simulink model "FullCarLateral"  (R2023b)
settings: Solver=FixedStepAuto  StartTime=0.0  StopTime=30  FixedStep=dt  MaxStep=0.001  RelTol=1e-3
model workspace (MAT data in the model file):
  AMU : Simulink.Signal (value not decoded)
  EPSILON : Simulink.Signal (value not decoded)
  FZO : Simulink.Signal (value not decoded)
  LCX : Simulink.Signal (value not decoded)
  LCY : Simulink.Signal (value not decoded)
  LCZ : Simulink.Signal (value not decoded)
  LEX : Simulink.Signal (value not decoded)
  LEY : Simulink.Signal (value not decoded)
  LFZO : Simulink.Signal (value not decoded)
  LHX : Simulink.Signal (value not decoded)
  LHY : Simulink.Signal (value not decoded)
  LKXKAPPA : Simulink.Signal (value not decoded)
  LKYALPHA : Simulink.Signal (value not decoded)
  LKYGAMMA : Simulink.Signal (value not decoded)
  LKZGAMMA : Simulink.Signal (value not decoded)
  LMR : Simulink.Signal (value not decoded)
  LMUV : Simulink.Signal (value not decoded)
  LMUX : Simulink.Signal (value not decoded)
  LMUXAST : Simulink.Signal (value not decoded)
  LMUXPRIME : Simulink.Signal (value not decoded)
  LMUY : Simulink.Signal (value not decoded)
  LMUYAST : Simulink.Signal (value not decoded)
  LMUYPRIME : Simulink.Signal (value not decoded)
  LMX : Simulink.Signal (value not decoded)
  LMY : Simulink.Signal (value not decoded)
  LS : Simulink.Signal (value not decoded)
  LT : Simulink.Signal (value not decoded)
  LVX : Simulink.Signal (value not decoded)
  LVY : Simulink.Signal (value not decoded)
  LVYKAPPA : Simulink.Signal (value not decoded)
  LXALPHA : Simulink.Signal (value not decoded)
  LYKAPPA : Simulink.Signal (value not decoded)
  PCX1 : Simulink.Signal (value not decoded)
  PCY1 : Simulink.Signal (value not decoded)
  PDX1 : Simulink.Signal (value not decoded)
  PDX2 : Simulink.Signal (value not decoded)
  PDX3 : Simulink.Signal (value not decoded)
  PDY1 : Simulink.Signal (value not decoded)
  PDY2 : Simulink.Signal (value not decoded)
  PDY3 : Simulink.Signal (value not decoded)
  PEX1 : Simulink.Signal (value not decoded)
  PEX2 : Simulink.Signal (value not decoded)
  PEX3 : Simulink.Signal (value not decoded)
  PEX4 : Simulink.Signal (value not decoded)
  PEY1 : Simulink.Signal (value not decoded)
  PEY2 : Simulink.Signal (value not decoded)
  PEY3 : Simulink.Signal (value not decoded)
  PEY4 : Simulink.Signal (value not decoded)
  PEY5 : Simulink.Signal (value not decoded)
  PHX1 : Simulink.Signal (value not decoded)
  PHX2 : Simulink.Signal (value not decoded)
  PHY1 : Simulink.Signal (value not decoded)
  PHY2 : Simulink.Signal (value not decoded)
  PKX1 : Simulink.Signal (value not decoded)
  PKX2 : Simulink.Signal (value not decoded)
  PKX3 : Simulink.Signal (value not decoded)
  PKY1 : Simulink.Signal (value not decoded)
  PKY2 : Simulink.Signal (value not decoded)
  PKY3 : Simulink.Signal (value not decoded)
  PKY4 : Simulink.Signal (value not decoded)
  PKY5 : Simulink.Signal (value not decoded)
  PKY6 : Simulink.Signal (value not decoded)
  PKY7 : Simulink.Signal (value not decoded)
  PVX1 : Simulink.Signal (value not decoded)
  PVX2 : Simulink.Signal (value not decoded)
  PVY1 : Simulink.Signal (value not decoded)
  PVY2 : Simulink.Signal (value not decoded)
  PVY3 : Simulink.Signal (value not decoded)
  PVY4 : Simulink.Signal (value not decoded)
  QBZ1 : Simulink.Signal (value not decoded)
  QBZ10 : Simulink.Signal (value not decoded)
  QBZ2 : Simulink.Signal (value not decoded)
  QBZ3 : Simulink.Signal (value not decoded)
  QBZ5 : Simulink.Signal (value not decoded)
  QBZ6 : Simulink.Signal (value not decoded)
  QBZ9 : Simulink.Signal (value not decoded)
  QCZ1 : Simulink.Signal (value not decoded)
  QDZ1 : Simulink.Signal (value not decoded)
  QDZ10 : Simulink.Signal (value not decoded)
  QDZ11 : Simulink.Signal (value not decoded)
  QDZ2 : Simulink.Signal (value not decoded)
  QDZ3 : Simulink.Signal (value not decoded)
  QDZ4 : Simulink.Signal (value not decoded)
  QDZ6 : Simulink.Signal (value not decoded)
  QDZ7 : Simulink.Signal (value not decoded)
  QDZ8 : Simulink.Signal (value not decoded)
  QDZ9 : Simulink.Signal (value not decoded)
  QEZ1 : Simulink.Signal (value not decoded)
  QEZ2 : Simulink.Signal (value not decoded)
  QEZ3 : Simulink.Signal (value not decoded)
  QEZ4 : Simulink.Signal (value not decoded)
  QEZ5 : Simulink.Signal (value not decoded)
  QHZ1 : Simulink.Signal (value not decoded)
  QHZ2 : Simulink.Signal (value not decoded)
  QHZ3 : Simulink.Signal (value not decoded)
  QHZ4 : Simulink.Signal (value not decoded)
  QSX1 : Simulink.Signal (value not decoded)
  QSX2 : Simulink.Signal (value not decoded)
  QSX3 : Simulink.Signal (value not decoded)
  QX1 : Simulink.Signal (value not decoded)
  QX2 : Simulink.Signal (value not decoded)
  QX3 : Simulink.Signal (value not decoded)
  QX4 : Simulink.Signal (value not decoded)
  QX5 : Simulink.Signal (value not decoded)
  QX6 : Simulink.Signal (value not decoded)
  RBX1 : Simulink.Signal (value not decoded)
  RBX2 : Simulink.Signal (value not decoded)
  RBX3 : Simulink.Signal (value not decoded)
  RBY1 : Simulink.Signal (value not decoded)
  RBY2 : Simulink.Signal (value not decoded)
  RBY3 : Simulink.Signal (value not decoded)
  RBY4 : Simulink.Signal (value not decoded)
  RCX1 : Simulink.Signal (value not decoded)
  RCY1 : Simulink.Signal (value not decoded)
  REX1 : Simulink.Signal (value not decoded)
  REX2 : Simulink.Signal (value not decoded)
  REY1 : Simulink.Signal (value not decoded)
  REY2 : Simulink.Signal (value not decoded)
  RHX1 : Simulink.Signal (value not decoded)
  RHY1 : Simulink.Signal (value not decoded)
  RHY2 : Simulink.Signal (value not decoded)
  RO : Simulink.Signal (value not decoded)
  RVY1 : Simulink.Signal (value not decoded)
  RVY2 : Simulink.Signal (value not decoded)
  RVY3 : Simulink.Signal (value not decoded)
  RVY4 : Simulink.Signal (value not decoded)
  RVY5 : Simulink.Signal (value not decoded)
  RVY6 : Simulink.Signal (value not decoded)
  SSZ1 : Simulink.Signal (value not decoded)
  SSZ2 : Simulink.Signal (value not decoded)
  SSZ3 : Simulink.Signal (value not decoded)
  SSZ4 : Simulink.Signal (value not decoded)
  VCX : Simulink.Signal (value not decoded)
  ZETA0 : Simulink.Signal (value not decoded)
  ZETA1 : Simulink.Signal (value not decoded)
  ZETA2 : Simulink.Signal (value not decoded)
  ZETA3 : Simulink.Signal (value not decoded)
  ZETA4 : Simulink.Signal (value not decoded)
  ZETA5 : Simulink.Signal (value not decoded)
  ZETA6 : Simulink.Signal (value not decoded)
  ZETA7 : Simulink.Signal (value not decoded)
  ZETA8 : Simulink.Signal (value not decoded)
values from neighbouring files (symbols this model uses):
  A = load('PSS LATERAL FORCE COEFFS.mat').A    [FullCarLateralParams.m]
  B = load('PSS ALIGNING TORQUE COEFFS.mat').B    [FullCarLateralParams.m]
  b = 0.085    [FullCarLateralParams.m]
  C = load('COMBINED OVERTURNING MOMENT COEFFS.mat').C    [FullCarLateralParams.m]
  c_roll = 0.1    [FullCarLateralParams.m]
  cD = 1.23    [FullCarLateralParams.m]
  cL = 3.71    [FullCarLateralParams.m]
  D = load('PLS LONGITUDINAL FORCE COEFFS.mat').D    [FullCarLateralParams.m]
  dt = 0.001    [FullCarLateralParams.m]
  E = load('COMBINED LONGITUDINAL FORCE COEFFS.mat').E    [FullCarLateralParams.m]
  e_FL = atan(tf/lf)    [FullCarLateralParams.m]
  e_FR = atan(lf/tf)    [FullCarLateralParams.m]
  e_RL = atan(lr/tr)    [FullCarLateralParams.m]
  e_RR = atan(tr/lr)    [FullCarLateralParams.m]
  F = load('COMBINED LATERAL FORCE COEFFS.mat').F    [FullCarLateralParams.m]
  frontalA = 1    [FullCarLateralParams.m]
  g = 9.81    [FullCarLateralParams.m]
  G = load('COMBINED ALIGNING TORQUE COEFFS.mat').G    [FullCarLateralParams.m]
  gearboxEff = 0.95    [FullCarLateralParams.m]
  GR = 11.86    [FullCarLateralParams.m]
  hCG = 0.2    [FullCarLateralParams.m]
  Ix_wheel = (0.07829 + Ix_motor*GR*GR) * Ix_wheel_factor    (= 0.1168307304)    [FullCarLateralParams.m]
  Iz_vehicle = 125    [FullCarLateralParams.m]
  lf = wb - lr    (= 0.755)    [FullCarLateralParams.m]
  lowpassT = 0.05    [FullCarLateralParams.m]
  lr = 0.78    [FullCarLateralParams.m]
  m = 250    [FullCarLateralParams.m]
  motorOmegaLimit = 2094    [FullCarLateralParams.m]
  R_FL = sqrt(tf^2 + lf^2)    [FullCarLateralParams.m]
  R_FR = R_FL    [FullCarLateralParams.m]
  R_RL = sqrt(tr^2 + lr^2)    [FullCarLateralParams.m]
  R_RR = R_RL    [FullCarLateralParams.m]
  R_wheel = 0.2    [FullCarLateralParams.m]
  rho = 1.293    [FullCarLateralParams.m]
  tireFactor_X_Accel = 0.6    [FullCarLateralParams.m]
  tireFactor_X_Brake = 0.6    [FullCarLateralParams.m]
  tireFactor_Y = 1    [FullCarLateralParams.m]
  TLLTD = 0.5    [FullCarLateralParams.m]
  tr = trackWidth / 2    (= 0.6)    [FullCarLateralParams.m]
  trackWidth = 1.2    [FullCarLateralParams.m]
  wb = 1.535    [FullCarLateralParams.m]
  wheelSideBrakeFactor = 1    [FullCarLateralParams.m]
undefined symbols (not defined in the file or in its folder): trackReference
libraries: simulink_extras x11, eeGeneralControl x3, slpidlib x2, simulink x2
(part 2 of 6)

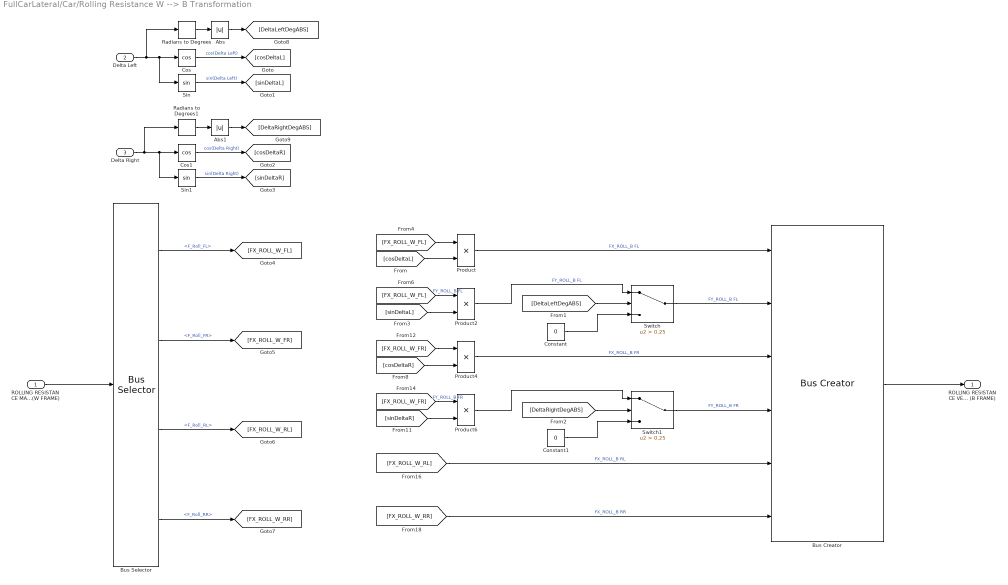
== system FullCarLateral/Car/Rolling Resistance W --> B Transformation ==
  ROLLING RESISTANCE MAGNITUDE (W FRAME) : Inport
  Delta Left : Inport  Port=2
  Delta Right : Inport  Port=3
  Abs : Abs  SaturateOnIntegerOverflow=off
  Abs1 : Abs  SaturateOnIntegerOverflow=off
  Bus Creator : BusCreator  Inputs=6
  Bus Selector : BusSelector  OutputSignals=F_Roll_FL,F_Roll_FR,F_Roll_RL,F_Roll_RR
  Constant : Constant  Value=0
  Constant1 : Constant  Value=0
  Cos : Trigonometry  Operator=cos
  Cos1 : Trigonometry  Operator=cos
  Product{,2,4,6} (4 alike) : Product
  Radians to Degrees : simulink_extras/Transformations/Radians to Degrees
  Radians to Degrees1 : simulink_extras/Transformations/Radians to Degrees
  Sin : Trigonometry
  Sin1 : Trigonometry
  Switch : Switch  Criteria=u2 > Threshold  Threshold=0.25  SaturateOnIntegerOverflow=off  InputSameDT=off
  Switch1 : Switch  Criteria=u2 > Threshold  Threshold=0.25  SaturateOnIntegerOverflow=off  InputSameDT=off
  ROLLING RESISTANCE VECTOR (B FRAME) : Outport
  wires:
  Bus Creator/1 -> ROLLING RESISTANCE VECTOR (B FRAME)/1
  [FX_ROLL_W_RR] -> Bus Creator/6  "FX_ROLL_B RR"
  [FX_ROLL_W_RL] -> Bus Creator/5  "FX_ROLL_B RL"
  [cosDeltaR] -> Product4/2
  Product4/1 -> Bus Creator/3  "FX_ROLL_B FR"
  [sinDeltaR] -> Product6/2
  [FX_ROLL_W_FR] -> Product4/1
  [FX_ROLL_W_FR] -> Product6/1  "FY_ROLL_B FR"
  [FX_ROLL_W_FL] -> Product2/1  "FY_ROLL_B FL"
  [FX_ROLL_W_FL] -> Product/1
  Bus Selector/4 -> [FX_ROLL_W_RR]  "<F_Roll_RR>"
  Bus Selector/3 -> [FX_ROLL_W_RL]  "<F_Roll_RL>"
  Bus Selector/2 -> [FX_ROLL_W_FR]  "<F_Roll_FR>"
  Bus Selector/1 -> [FX_ROLL_W_FL]  "<F_Roll_FL>"
  [sinDeltaL] -> Product2/2
  Product/1 -> Bus Creator/1  "FX_ROLL_B FL"
  [cosDeltaL] -> Product/2
  Cos1/1 -> [cosDeltaR]  "cos(Delta Right)"
  Sin1/1 -> [sinDeltaR]  "sin(Delta Right)"
  Sin/1 -> [sinDeltaL]  "sin(Delta Left)"
  Cos/1 -> [cosDeltaL]  "cos(Delta Left)"
  Delta Left/1 -> Radians to Degrees/1, Cos/1, Sin/1
  ROLLING RESISTANCE MAGNITUDE (W FRAME)/1 -> Bus Selector/1
  Radians to Degrees/1 -> Abs/1
  Radians to Degrees1/1 -> Abs1/1
  Delta Right/1 -> Radians to Degrees1/1, Sin1/1, Cos1/1
  Abs/1 -> [DeltaLeftDegABS]
  Abs1/1 -> [DeltaRightDegABS]
  [DeltaLeftDegABS] -> Switch/2
  Constant/1 -> Switch/3
  Product2/1 -> Switch/1  "FY_ROLL_B FL"
  [DeltaRightDegABS] -> Switch1/2
  Constant1/1 -> Switch1/3
  Product6/1 -> Switch1/1
  Switch/1 -> Bus Creator/2  "FY_ROLL_B FL"
  Switch1/1 -> Bus Creator/4  "FY_ROLL_B FR"

== system FullCarLateral/Car/Slip Angle and Corner Velocity ==
  Vx_B : Inport
  Vy_B : Inport  Port=2
  Yaw Rate : Inport  Port=3
  Delta Left : Inport  Port=4
  Delta Right : Inport  Port=5
  Bus Creator : BusCreator  Inputs=4
  Bus Creator1 : BusCreator  Inputs=4
  Constant : Constant  Value=R_FL
  Constant1 : Constant  Value=R_FR
  Constant2 : Constant  Value=R_RL
  Constant3 : Constant  Value=R_RR
  Constant4 : Constant  Value=e_FL
  Constant5 : Constant  Value=e_FR
  Constant6 : Constant  Value=e_RL
  Constant7 : Constant  Value=e_RR
  MATLAB Function : MATLAB Function  TreatAsAtomicUnit=on
  Alpha : Outport
  LONGITUDINAL CORNER VEL (DIRECTION OF BODY) : Outport  Port=2
  wires:
  Constant3/1 -> MATLAB Function/9(R_RR)
  Bus Creator1/1 -> LONGITUDINAL CORNER VEL (DIRECTION OF BODY)/1
  Constant7/1 -> MATLAB Function/13(e_RR)
  Constant2/1 -> MATLAB Function/8(R_RL)
  MATLAB Function/5(LongCornerVel_FL_B) -> Bus Creator1/1
  Constant4/1 -> MATLAB Function/10(e_FL)
  Constant/1 -> MATLAB Function/6(R_FL)
  Bus Creator/1 -> Alpha/1
  MATLAB Function/7(LongCornerVel_RL_B) -> Bus Creator1/3
  MATLAB Function/8(LongCornerVel_RR_B) -> Bus Creator1/4
  MATLAB Function/6(LongCornerVel_FR_B) -> Bus Creator1/2
  Constant6/1 -> MATLAB Function/12(e_RL)
  Constant5/1 -> MATLAB Function/11(e_FR)
  Vx_B/1 -> MATLAB Function/1(Vx_B)
  Vy_B/1 -> MATLAB Function/2(Vy_B)
  Yaw Rate/1 -> MATLAB Function/3(Yaw_Rate)
  Delta Left/1 -> MATLAB Function/4(Delta_Left)
  Delta Right/1 -> MATLAB Function/5(Delta_Right)
  Constant1/1 -> MATLAB Function/7(R_FR)
  MATLAB Function/1(Alpha_FL) -> Bus Creator/1  "Alpha_FL"
  MATLAB Function/2(Alpha_FR) -> Bus Creator/2  "Alpha_FR"
  MATLAB Function/3(Alpha_RL) -> Bus Creator/3  "Alpha_RL"
  MATLAB Function/4(Alpha_RR) -> Bus Creator/4  "Alpha_RR"

== system FullCarLateral/Car/Steering Kinematics ==
  Delta Avg (DEG) : Inport
  Abs : Abs  SaturateOnIntegerOverflow=off
  Abs1 : Abs  SaturateOnIntegerOverflow=off
  Ackerman Calculation : Subsystem  TreatAsAtomicUnit=on
  Constant : Constant  Value=0
  Constant1 : Constant  Value=0
  Degrees to Radians : simulink_extras/Transformations/Degrees to Radians
  If : If  IfExpression=u1 ~= 0  ShowElse=off
  Switch : Switch  Criteria=u2 > Threshold  SaturateOnIntegerOverflow=off  InputSameDT=off
  Switch1 : Switch  Criteria=u2 > Threshold  SaturateOnIntegerOverflow=off  InputSameDT=off
  Delta Left : Outport
  Delta Right : Outport  Port=2
  wires:
  Constant1/1 -> Switch/3
  Constant/1 -> Switch1/3
  Delta Avg (DEG)/1 -> Degrees to Radians/1, Abs1/1, Abs/1, Ackerman Calculation/1(Delta Avg), If/1
  If/1 -> Ackerman Calculation/Action
  Abs/1 -> Switch/2
  Abs1/1 -> Switch1/2
  Switch/1 -> Delta Left/1
  Switch1/1 -> Delta Right/1
  Degrees to Radians/1 -> Switch1/1, Switch/1

== system FullCarLateral/Car/Subsystem ==
  Speed : Inport
  Fcn4 : Fcn  Expr=0.5*(u*u)*rho*frontalA*cD
  DRAG FORCE MAGNITUDE : Outport
  wires:
  Speed/1 -> Fcn4/1
  Fcn4/1 -> DRAG FORCE MAGNITUDE/1

== system FullCarLateral/Car/Subsystem1 ==
  Ax_B : Inport
  Ay_B : Inport  Port=2
  Vx_B : Inport  Port=3
  Vy_B : Inport  Port=4
  Yaw_Accel : Inport  Port=5
  Yaw_Rate : Inport  Port=6
  Speed : Inport  Port=7
  Bus Creator2 : BusCreator  Inputs=7
  To Workspace2 : ToWorkspace  VariableName=bFrame  SaveFormat=Timeseries  SampleTime=-1
  wires:
  Yaw_Accel/1 -> Bus Creator2/5
  Bus Creator2/1 -> To Workspace2/1
  Yaw_Rate/1 -> Bus Creator2/6
  Vx_B/1 -> Bus Creator2/2
  Vy_B/1 -> Bus Creator2/4
  Speed/1 -> Bus Creator2/7
  Ay_B/1 -> Bus Creator2/3
  Ax_B/1 -> Bus Creator2/1

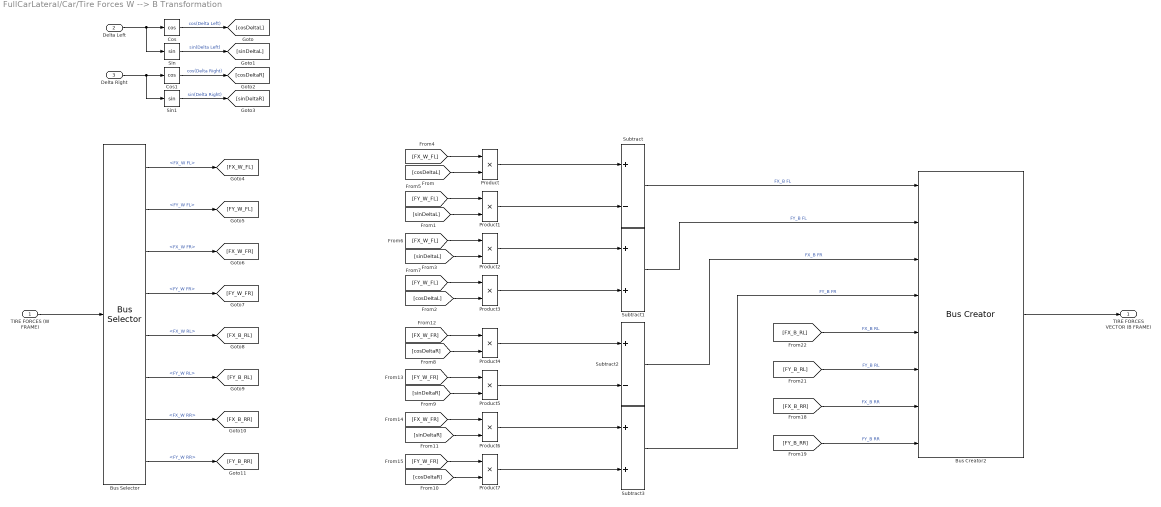
== system FullCarLateral/Car/Tire Forces W --> B Transformation ==
  TIRE FORCES (W FRAME) : Inport
  Delta Left : Inport  Port=2
  Delta Right : Inport  Port=3
  Bus Creator2 : BusCreator  Inputs=8
  Bus Selector : BusSelector  OutputSignals=FX_W FL,FY_W FL,FX_W FR,FY_W FR,FX_W RL,FY_W RL,FX_W RR,FY_W RR
  Cos : Trigonometry  Operator=cos
  Cos1 : Trigonometry  Operator=cos
  Product{,1..7} (8 alike) : Product
  Sin : Trigonometry
  Sin1 : Trigonometry
  Subtract : Sum  Inputs=+-
  Subtract1 : Sum
  Subtract2 : Sum  Inputs=+-
  Subtract3 : Sum
  TIRE FORCES VECTOR (B FRAME) : Outport
  wires:
  TIRE FORCES (W FRAME)/1 -> Bus Selector/1
  Delta Left/1 -> Sin/1, Cos/1
  Cos/1 -> [cosDeltaL]  "cos(Delta Left)"
  Sin/1 -> [sinDeltaL]  "sin(Delta Left)"
  Sin1/1 -> [sinDeltaR]  "sin(Delta Right)"
  Cos1/1 -> [cosDeltaR]  "cos(Delta Right)"
  Delta Right/1 -> Cos1/1, Sin1/1
  [cosDeltaL] -> Product/2
  Product/1 -> Subtract/1
  [sinDeltaL] -> Product1/2
  Product1/1 -> Subtract/2
  Subtract1/1 -> Bus Creator2/2  "FY_B FL"
  Product3/1 -> Subtract1/2
  Product2/1 -> Subtract1/1
  [sinDeltaL] -> Product2/2
  [cosDeltaL] -> Product3/2
  Bus Selector/1 -> [FX_W_FL]  "<FX_W FL>"
  Bus Selector/2 -> [FY_W_FL]  "<FY_W FL>"
  Bus Selector/3 -> [FX_W_FR]  "<FX_W FR>"
  Bus Selector/4 -> [FY_W_FR]  "<FY_W FR>"
  [FX_W_FL] -> Product/1
  [FY_W_FL] -> Product1/1
  [FX_W_FL] -> Product2/1
  [FY_W_FL] -> Product3/1
  [FY_W_FR] -> Product7/1
  [FX_W_FR] -> Product6/1
  [FY_W_FR] -> Product5/1
  [FX_W_FR] -> Product4/1
  [cosDeltaR] -> Product7/2
  [sinDeltaR] -> Product6/2
  Product6/1 -> Subtract3/1
  Product7/1 -> Subtract3/2
  Subtract3/1 -> Bus Creator2/4  "FY_B FR"
  Subtract2/1 -> Bus Creator2/3  "FX_B FR"
  Product5/1 -> Subtract2/2
  [sinDeltaR] -> Product5/2
  Product4/1 -> Subtract2/1
  [cosDeltaR] -> Product4/2
  Bus Selector/5 -> [FX_B_RL]  "<FX_W RL>"
  Bus Selector/6 -> [FY_B_RL]  "<FY_W RL>"
  Bus Selector/7 -> [FX_B_RR]  "<FX_W RR>"
  Bus Selector/8 -> [FY_B_RR]  "<FY_W RR>"
  [FX_B_RR] -> Bus Creator2/7  "FX_B RR"
  [FY_B_RR] -> Bus Creator2/8  "FY_B RR"
  Subtract/1 -> Bus Creator2/1  "FX_B FL"
  [FY_B_RL] -> Bus Creator2/6  "FY_B RL"
  [FX_B_RL] -> Bus Creator2/5  "FX_B RL"
  Bus Creator2/1 -> TIRE FORCES VECTOR (B FRAME)/1

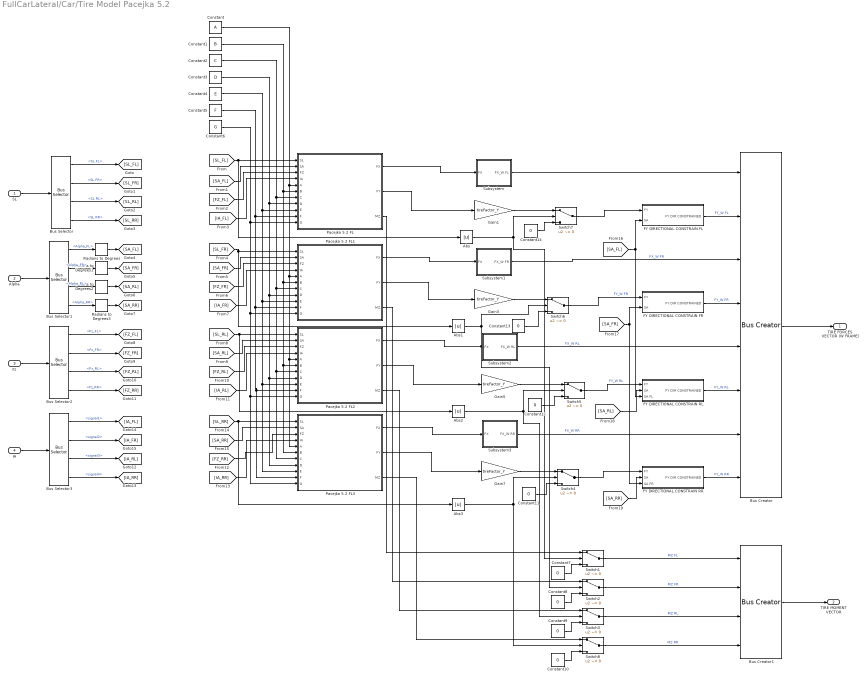
== system FullCarLateral/Car/Tire Model Pacejka 5.2 ==
  SL : Inport
  Alpha : Inport  Port=2
  Fz : Inport  Port=3
  IA : Inport  Port=4
  Abs{,1..3} (4 alike) : Abs  SaturateOnIntegerOverflow=off
  Bus Creator : BusCreator  Inputs=8
  Bus Creator1 : BusCreator  Inputs=4
  Bus Selector : BusSelector  OutputSignals=SL FL,SL FR,SL RL,SL RR
  Bus Selector1 : BusSelector  OutputSignals=Alpha_FL,Alpha_FR,Alpha_RL,Alpha_RR
  Bus Selector2 : BusSelector  OutputSignals=Fz_FL,Fz_FR,Fz_RL,Fz_RR
  Bus Selector3 : BusSelector  OutputSignals=signal1,signal2,signal3,signal4
  Constant : Constant  Value=A
  Constant1 : Constant  Value=B
  Constant{7..14} (8 alike) : Constant  Value=0
  Constant2 : Constant  Value=C
  Constant3 : Constant  Value=D
  Constant4 : Constant  Value=E
  Constant5 : Constant  Value=F
  Constant6 : Constant  Value=G
  FY DIRECTIONAL CONSTRAIN FL : Subsystem
  FY DIRECTIONAL CONSTRAIN FR : Subsystem
  FY DIRECTIONAL CONSTRAIN RL : Subsystem
  FY DIRECTIONAL CONSTRAIN RR : Subsystem
  Gain{1,3,5,7} (4 alike) : Gain  Gain=tireFactor_Y
  Pacejka 5.2 FL : MATLAB Function  TreatAsAtomicUnit=on  SystemSampleTime=dt
  Pacejka 5.2 FL1 : MATLAB Function  TreatAsAtomicUnit=on  SystemSampleTime=dt
  Pacejka 5.2 FL2 : MATLAB Function  TreatAsAtomicUnit=on  SystemSampleTime=dt
  Pacejka 5.2 FL3 : MATLAB Function  TreatAsAtomicUnit=on  SystemSampleTime=dt
  Radians to Degrees{,1..3} (4 alike) : simulink_extras/Transformations/Radians to Degrees
  Subsystem : Subsystem
  Subsystem1 : Subsystem
  Subsystem2 : Subsystem
  Subsystem3 : Subsystem
  Switch{1..8} (8 alike) : Switch  Criteria=u2 ~= 0  SaturateOnIntegerOverflow=off  InputSameDT=off
  TIRE FORCES VECTOR (W FRAME) : Outport
  TIRE MOMENT VECTOR : Outport  Port=2
  wires:
  Bus Selector2/2 -> [FZ_FR]  "<Fz_FR>"
  Bus Selector/4 -> [SL_RR]  "<SL RR>"
  Bus Creator/1 -> TIRE FORCES VECTOR (W FRAME)/1
  Alpha/1 -> Bus Selector1/1
  [SL_FR] -> Abs1/1, Pacejka 5.2 FL1/1(SL)
  Fz/1 -> Bus Selector2/1
  Bus Selector1/4 -> Radians to Degrees3/1  "<Alpha_RR>"
  SL/1 -> Bus Selector/1
  [SL_FL] -> Abs/1, Pacejka 5.2 FL/1(SL)
  Bus Selector1/3 -> Radians to Degrees2/1  "<Alpha_RL>"
  Bus Selector1/1 -> Radians to Degrees/1  "<Alpha_FL>"
  Bus Selector2/1 -> [FZ_FL]  "<Fz_FL>"
  Bus Selector2/4 -> [FZ_RR]  "<Fz_RR>"
  [FZ_FL] -> Pacejka 5.2 FL/3(FZ)
  Bus Selector1/2 -> Radians to Degrees1/1  "<Alpha_FR>"
  [IA_FL] -> Pacejka 5.2 FL/4(IA)
  Bus Selector3/3 -> [IA_RL]  "<signal3>"
  Bus Selector/1 -> [SL_FL]  "<SL FL>"
  Bus Selector3/2 -> [IA_FR]  "<signal2>"
  Bus Selector3/4 -> [IA_RR]  "<signal4>"
  Bus Selector/3 -> [SL_RL]  "<SL RL>"
  IA/1 -> Bus Selector3/1
  Bus Selector3/1 -> [IA_FL]  "<signal1>"
  [SA_FL] -> Pacejka 5.2 FL/2(SA)
  Bus Selector2/3 -> [FZ_RL]  "<Fz_RL>"
  Bus Selector/2 -> [SL_FR]  "<SL FR>"
  Constant/1 -> Pacejka 5.2 FL1/5(A), Pacejka 5.2 FL3/5(A), Pacejka 5.2 FL2/5(A), Pacejka 5.2 FL/5(A)
  Constant1/1 -> Pacejka 5.2 FL1/6(B), Pacejka 5.2 FL3/6(B), Pacejka 5.2 FL2/6(B), Pacejka 5.2 FL/6(B)
  Constant2/1 -> Pacejka 5.2 FL1/7(C), Pacejka 5.2 FL3/7(C), Pacejka 5.2 FL2/7(C), Pacejka 5.2 FL/7(C)
  Constant3/1 -> Pacejka 5.2 FL1/8(D), Pacejka 5.2 FL3/8(D), Pacejka 5.2 FL2/8(D), Pacejka 5.2 FL/8(D)
  Constant4/1 -> Pacejka 5.2 FL1/9(E), Pacejka 5.2 FL3/9(E), Pacejka 5.2 FL2/9(E), Pacejka 5.2 FL/9(E)
  Constant5/1 -> Pacejka 5.2 FL1/10(F), Pacejka 5.2 FL3/10(F), Pacejka 5.2 FL2/10(F), Pacejka 5.2 FL/10(F)
  Constant6/1 -> Pacejka 5.2 FL1/11(G), Pacejka 5.2 FL3/11(G), Pacejka 5.2 FL2/11(G), Pacejka 5.2 FL/11(G)
  [SA_FR] -> Pacejka 5.2 FL1/2(SA)
  [FZ_FR] -> Pacejka 5.2 FL1/3(FZ)
  [IA_FR] -> Pacejka 5.2 FL1/4(IA)
  [SL_RR] -> Pacejka 5.2 FL3/1(SL), Abs3/1
  [SA_RR] -> Pacejka 5.2 FL3/2(SA)
  [FZ_RR] -> Pacejka 5.2 FL3/3(FZ)
  [IA_RR] -> Pacejka 5.2 FL3/4(IA)
  [SL_RL] -> Pacejka 5.2 FL2/1(SL), Abs2/1
  [SA_RL] -> Pacejka 5.2 FL2/2(SA)
  [FZ_RL] -> Pacejka 5.2 FL2/3(FZ)
  [IA_RL] -> Pacejka 5.2 FL2/4(IA)
  Subsystem1/1(FX_W FR) -> Bus Creator/3  "FX_W FR"
  Subsystem2/1(FX_W RL) -> Bus Creator/5  "FX_W RL"
  Subsystem3/1(FX_W RR) -> Bus Creator/7  "FX_W RR"
  Radians to Degrees/1 -> [SA_FL]
  Radians to Degrees1/1 -> [SA_FR]
  Radians to Degrees2/1 -> [SA_RL]
  Radians to Degrees3/1 -> [SA_RR]
  FY DIRECTIONAL CONSTRAIN FL/1(FY DIR CONSTRAINED) -> Bus Creator/2  "FY_W FL"
  [SA_FL] -> FY DIRECTIONAL CONSTRAIN FL/2(SA), FY DIRECTIONAL CONSTRAIN RL/3(SA FL)
  FY DIRECTIONAL CONSTRAIN FR/1(FY DIR CONSTRAINED) -> Bus Creator/4  "FY_W FR"
  [SA_FR] -> FY DIRECTIONAL CONSTRAIN RR/3(SA FR), FY DIRECTIONAL CONSTRAIN FR/2(SA)
  [SA_RL] -> FY DIRECTIONAL CONSTRAIN RL/2(SA)
  FY DIRECTIONAL CONSTRAIN RL/1(FY DIR CONSTRAINED) -> Bus Creator/6  "FY_W RL"
  [SA_RR] -> FY DIRECTIONAL CONSTRAIN RR/2(SA)
  FY DIRECTIONAL CONSTRAIN RR/1(FY DIR CONSTRAINED) -> Bus Creator/8  "FY_W RR"
  Subsystem/1(FX_W FL) -> Bus Creator/1
  Gain7/1 -> Switch4/1
  Constant11/1 -> Switch4/3
  Gain5/1 -> Switch5/1
  Constant12/1 -> Switch5/3
  Gain3/1 -> Switch6/1
  Constant13/1 -> Switch6/3
  Gain1/1 -> Switch7/1
  Constant14/1 -> Switch7/3
  Abs/1 -> Switch1/2, Switch7/2
  Switch7/1 -> FY DIRECTIONAL CONSTRAIN FL/1(FY)
  Switch6/1 -> FY DIRECTIONAL CONSTRAIN FR/1(FY)  "FY_W FR"
  Abs1/1 -> Switch6/2, Switch2/2
  Abs2/1 -> Switch3/2, Switch5/2
  Switch4/1 -> FY DIRECTIONAL CONSTRAIN RR/1(FY)
  Abs3/1 -> Switch8/2, Switch4/2
  Switch5/1 -> FY DIRECTIONAL CONSTRAIN RL/1(FY)  "FY_W RL"
  Pacejka 5.2 FL/1(FX) -> Subsystem/1(FX)
  Pacejka 5.2 FL/2(FY) -> Gain1/1
  Pacejka 5.2 FL1/1(FX) -> Subsystem1/1(FX)
  Pacejka 5.2 FL1/2(FY) -> Gain3/1
  Pacejka 5.2 FL2/1(FX) -> Subsystem2/1(FX)
  Pacejka 5.2 FL2/2(FY) -> Gain5/1
  Pacejka 5.2 FL3/1(FX) -> Subsystem3/1(FX)
  Pacejka 5.2 FL3/2(FY) -> Gain7/1
  Bus Creator1/1 -> TIRE MOMENT VECTOR/1
  Constant7/1 -> Switch1/3
  Switch1/1 -> Bus Creator1/1  "MZ FL"
  Constant8/1 -> Switch2/3
  Constant9/1 -> Switch3/3
  Constant10/1 -> Switch8/3
  Switch8/1 -> Bus Creator1/4  "MZ RR"
  Switch3/1 -> Bus Creator1/3  "MZ RL"
  Switch2/1 -> Bus Creator1/2  "MZ FR"
  Pacejka 5.2 FL3/3(MZ) -> Switch8/1
  Pacejka 5.2 FL2/3(MZ) -> Switch3/1
  Pacejka 5.2 FL1/3(MZ) -> Switch2/1
  Pacejka 5.2 FL/3(MZ) -> Switch1/1

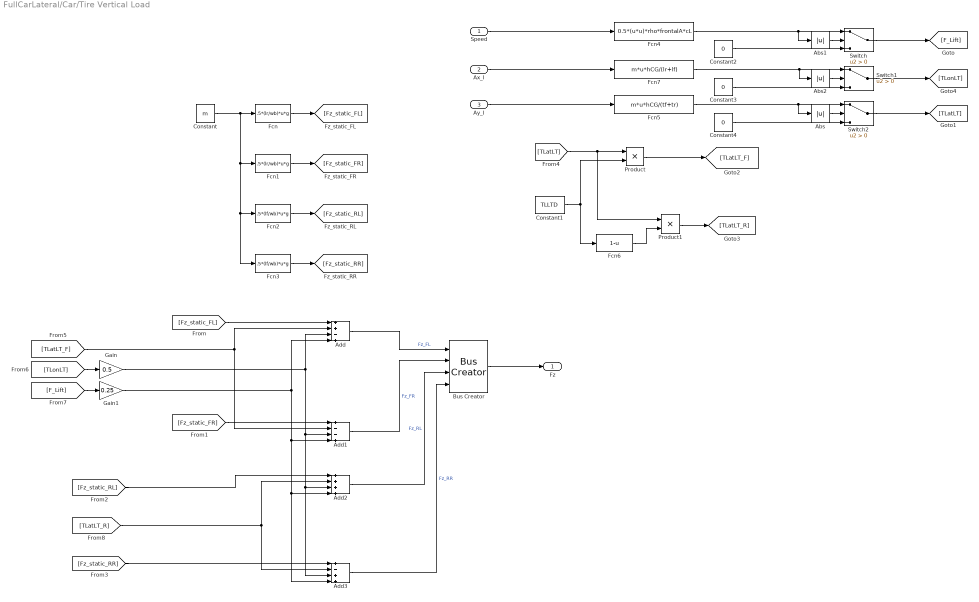
== system FullCarLateral/Car/Tire Vertical Load ==
  Speed : Inport
  Ax_I : Inport  Port=2
  Ay_I : Inport  Port=3
  Abs : Abs  SaturateOnIntegerOverflow=off
  Abs1 : Abs  SaturateOnIntegerOverflow=off
  Abs2 : Abs  SaturateOnIntegerOverflow=off
  Add : Sum  Inputs=++-+
  Add1 : Sum  Inputs=+--+
  Add2 : Sum  Inputs=++++
  Add3 : Sum  Inputs=+-++
  Bus Creator : BusCreator  Inputs=4
  Constant : Constant  Value=m
  Constant1 : Constant  Value=TLLTD
  Constant2 : Constant  Value=0
  Constant3 : Constant  Value=0
  Constant4 : Constant  Value=0
  Fcn : Fcn  Expr=.5*(lr/wb)*u*g
  Fcn1 : Fcn  Expr=.5*(lr/wb)*u*g
  Fcn2 : Fcn  Expr=.5*(lf/wb)*u*g
  Fcn3 : Fcn  Expr=.5*(lf/wb)*u*g
  Fcn4 : Fcn  Expr=0.5*(u*u)*rho*frontalA*cL
  Fcn5 : Fcn  Expr=m*u*hCG/(tf+tr)
  Fcn6 : Fcn  Expr=1-u
  Fcn7 : Fcn  Expr=m*u*hCG/(lr+lf)
  Gain : Gain  Gain=0.5
  Gain1 : Gain  Gain=0.25
  Product : Product
  Product1 : Product
  Switch : Switch  Criteria=u2 > Threshold  SaturateOnIntegerOverflow=off  InputSameDT=off
  Switch1 : Switch  Criteria=u2 > Threshold  SaturateOnIntegerOverflow=off  InputSameDT=off
  Switch2 : Switch  Criteria=u2 > Threshold  SaturateOnIntegerOverflow=off  InputSameDT=off
  Fz : Outport
  wires:
  Constant/1 -> Fcn3/1, Fcn2/1, Fcn1/1, Fcn/1
  Fcn/1 -> [Fz_static_FL]
  Fcn1/1 -> [Fz_static_FR]
  Fcn3/1 -> [Fz_static_RR]
  Fcn2/1 -> [Fz_static_RL]
  Bus Creator/1 -> Fz/1
  Speed/1 -> Fcn4/1
  Ay_I/1 -> Fcn5/1
  [TLatLT] -> Product1/1, Product/1
  Constant1/1 -> Fcn6/1, Product/2
  Product/1 -> [TLatLT_F]
  Fcn6/1 -> Product1/2
  Product1/1 -> [TLatLT_R]
  Ax_I/1 -> Fcn7/1
  [Fz_static_FL] -> Add/1
  [TLatLT_F] -> Add1/2, Add/2
  [TLonLT] -> Gain/1
  Gain/1 -> Add3/3, Add2/3, Add1/3, Add/3
  [F_Lift] -> Gain1/1
  Gain1/1 -> Add3/4, Add2/4, Add1/4, Add/4
  Add/1 -> Bus Creator/1  "Fz_FL"
  [Fz_static_FR] -> Add1/1
  Add1/1 -> Bus Creator/2  "Fz_FR"
  [Fz_static_RL] -> Add2/1
  [TLatLT_R] -> Add3/2, Add2/2
  Add2/1 -> Bus Creator/3  "Fz_RL"
  [Fz_static_RR] -> Add3/1
  Add3/1 -> Bus Creator/4  "Fz_RR"
  Fcn4/1 -> Switch/1, Abs1/1
  Switch/1 -> [F_Lift]
  Constant2/1 -> Switch/3
  Switch1/1 -> [TLonLT]
  Fcn7/1 -> Switch1/1, Abs2/1
  Constant3/1 -> Switch1/3
  Switch2/1 -> [TLatLT]
  Fcn5/1 -> Switch2/1, Abs/1
  Constant4/1 -> Switch2/3
  Abs/1 -> Switch2/2
  Abs1/1 -> Switch/2
  Abs2/1 -> Switch1/2

== system FullCarLateral/Car/Velocity B --> Velocity I Transformation ==
  dXdt_B : Inport  Unit=m/s
  dYdt_B : Inport  Port=2  Unit=m/s
  dYawdt : Inport  Port=3  Unit=rad/s
  Body Slip (RAD) : Inport  Port=4
  Add : Sum
  Add1 : Sum
  Add3 : Sum
  Constant6 : Constant  Value=dt
  Cos1 : Trigonometry  Operator=cos
  Data Store Memory2 : DataStoreMemory  DataStoreName=YAW_ANGLE  WriteAfterWriteMsg=warning  ShowAdditionalParam=off
  Data Store Read2 : DataStoreRead  DataStoreName=YAW_ANGLE  IndexOptions=Index vector (dialog)  Indices=1  OutputSizes=1
  Data Store Write2 : DataStoreWrite  DataStoreName=YAW_ANGLE  IndexOptions=Index vector (dialog)  Indices=1  OutputSizes=1
  Memory2 : Memory
  Product{2..6} (5 alike) : Product
  Sin1 : Trigonometry
  Subtract : Sum  Inputs=+-
  dXdt_Inertial : Outport
  dYdt_Inertial : Outport  Port=2
  YAW ANGLE : Outport  Port=3  Unit=rad
  wires:
  Data Store Read2/1 -> Add3/2
  Constant6/1 -> Product2/2
  Product2/1 -> Add3/1  "dYaw"
  Add3/1 -> Memory2/1
  dYawdt/1 -> Product2/1
  Product3/1 -> Add/1
  [cosYawBeta] -> Product4/2, Product5/2
  Product4/1 -> Subtract/1
  Product6/1 -> Subtract/2
  dXdt_B/1 -> Product4/1, Product3/1
  Subtract/1 -> dXdt_Inertial/1
  Add/1 -> dYdt_Inertial/1
  [sinYawBeta] -> Product3/2, Product6/2
  Product5/1 -> Add/2
  dYdt_B/1 -> Product6/1, Product5/1
  Cos1/1 -> [cosYawBeta]  "cos(Yaw + Beta)"
  Memory2/1 -> Add1/1, YAW ANGLE/1, Data Store Write2/1
  Sin1/1 -> [sinYawBeta]  "sin(Yaw + Beta)"
  Add1/1 -> Sin1/1, Cos1/1
  Body Slip (RAD)/1 -> Add1/2

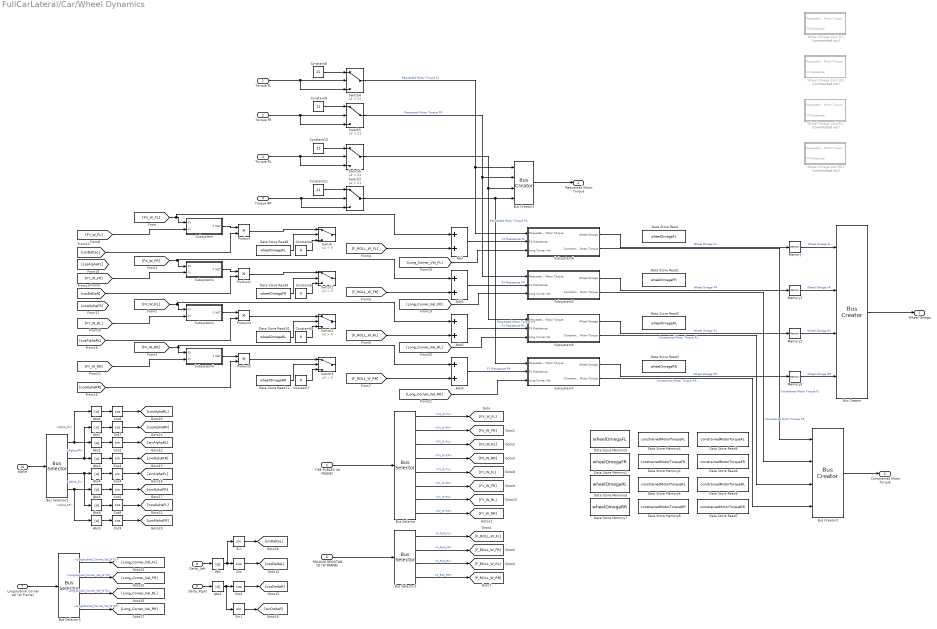
== system FullCarLateral/Car/Wheel Dynamics ==
  Torque FL : Inport
  Torque FR : Inport  Port=2
  Torque RL : Inport  Port=3
  Torque RR : Inport  Port=4
  TIRE FORCES (W FRAME) : Inport  Port=5
  ROLLING RESISTANCE (W FRAME) : Inport  Port=6
  Longitudinal Corner Vel (W Frame) : Inport  Port=7
  Delta_Left : Inport  Port=8
  Delta_Right : Inport  Port=9
  Alpha : Inport  Port=10
  Abs{,1..9} (10 alike) : Abs  SaturateOnIntegerOverflow=off
  Add{,1..3} (4 alike) : Sum
  Bus Creator : BusCreator  Inputs=4
  Bus Creator1 : BusCreator  Inputs=4
  Bus Creator2 : BusCreator  Inputs=4
  Bus Selector : BusSelector  OutputSignals=FX_W FL,FX_W FR,FX_W RL,FX_W RR,FY_W FL,FY_W FR,FY_W RL,FY_W RR
  Bus Selector1 : BusSelector  OutputSignals=F_Roll_FL,F_Roll_FR,F_Roll_RL,F_Roll_RR
  Bus Selector2 : BusSelector  OutputSignals=Alpha_RL,Alpha_RR,Alpha_FL,Alpha_FR
  Bus Selector3 : BusSelector  OutputSignals=Longitudinal_Corner_Vel_W FL,Longitudinal_Corner_Vel_W FR,Longitudinal_Corner_Vel_W RL,Longtidutinal_Corner_Vel_W RR
  Constant{8..11} (4 alike) : Constant  Value=21
  Constant{4..7} (4 alike) : Constant  Value=0
  Cos{,1,6..9} (6 alike) : Trigonometry  Operator=cos
  Cos{2..5} (4 alike) : Trigonometry
  Data Store Memory1 : DataStoreMemory  DataStoreName=wheelOmegaFR  WriteAfterWriteMsg=warning  ShowAdditionalParam=off
  Data Store Memory2 : DataStoreMemory  DataStoreName=constrainedMotorTorqueFR  WriteAfterWriteMsg=warning  ShowAdditionalParam=off
  Data Store Memory3 : DataStoreMemory  DataStoreName=wheelOmegaFL  WriteAfterWriteMsg=warning  ShowAdditionalParam=off
  Data Store Memory4 : DataStoreMemory  DataStoreName=constrainedMotorTorqueFL  WriteAfterWriteMsg=warning  ShowAdditionalParam=off
  Data Store Memory5 : DataStoreMemory  DataStoreName=wheelOmegaRL  WriteAfterWriteMsg=warning  ShowAdditionalParam=off
  Data Store Memory6 : DataStoreMemory  DataStoreName=constrainedMotorTorqueRL  WriteAfterWriteMsg=warning  ShowAdditionalParam=off
  Data Store Memory7 : DataStoreMemory  DataStoreName=wheelOmegaRR  WriteAfterWriteMsg=warning  ShowAdditionalParam=off
  Data Store Memory8 : DataStoreMemory  DataStoreName=constrainedMotorTorqueRR  WriteAfterWriteMsg=warning  ShowAdditionalParam=off
  Data Store Read : DataStoreRead  DataStoreName=wheelOmegaFL  IndexOptions=Index vector (dialog)  Indices=1  OutputSizes=1
  Data Store Read1 : DataStoreRead  DataStoreName=wheelOmegaFR  IndexOptions=Index vector (dialog)  Indices=1  OutputSizes=1
  Data Store Read10 : DataStoreRead  DataStoreName=wheelOmegaRL  IndexOptions=Index vector (dialog)  Indices=1  OutputSizes=1
  Data Store Read11 : DataStoreRead  DataStoreName=wheelOmegaRR  IndexOptions=Index vector (dialog)  Indices=1  OutputSizes=1
  Data Store Read2 : DataStoreRead  DataStoreName=wheelOmegaRL  IndexOptions=Index vector (dialog)  Indices=1  OutputSizes=1
  Data Store Read3 : DataStoreRead  DataStoreName=wheelOmegaRR  IndexOptions=Index vector (dialog)  Indices=1  OutputSizes=1
  Data Store Read4 : DataStoreRead  DataStoreName=constrainedMotorTorqueFR  IndexOptions=Index vector (dialog)  Indices=1  OutputSizes=1
  Data Store Read5 : DataStoreRead  DataStoreName=constrainedMotorTorqueRL  IndexOptions=Index vector (dialog)  Indices=1  OutputSizes=1
  Data Store Read6 : DataStoreRead  DataStoreName=constrainedMotorTorqueFL  IndexOptions=Index vector (dialog)  Indices=1  OutputSizes=1
  Data Store Read7 : DataStoreRead  DataStoreName=constrainedMotorTorqueRR  IndexOptions=Index vector (dialog)  Indices=1  OutputSizes=1
  Data Store Read8 : DataStoreRead  DataStoreName=wheelOmegaFL  IndexOptions=Index vector (dialog)  Indices=1  OutputSizes=1
  Data Store Read9 : DataStoreRead  DataStoreName=wheelOmegaFR  IndexOptions=Index vector (dialog)  Indices=1  OutputSizes=1
  Memory{,1..3} (4 alike) : Memory
  Product{,1..3} (4 alike) : Product
  Sin : Trigonometry
  Sin1 : Trigonometry
  Subsystem : Subsystem
  Subsystem1 : Subsystem
  Subsystem2 : Subsystem
  Subsystem3 : Subsystem
  Subsystem4 : Subsystem
  Subsystem5 : Subsystem
  Subsystem6 : Subsystem
  Subsystem7 : Subsystem
  Switch{,1..3} (4 alike) : Switch  Criteria=u2 > Threshold  SaturateOnIntegerOverflow=off  InputSameDT=off
  Switch{4..7} (4 alike) : Switch  Criteria=u2 > Threshold  Threshold=21  SaturateOnIntegerOverflow=off  InputSameDT=off
  Wheel Omega Calc FL1 : Subsystem  Commented=on
  Wheel Omega Calc FR1 : Subsystem  Commented=on
  Wheel Omega Calc RL1 : Subsystem  Commented=on
  Wheel Omega Calc RR1 : Subsystem  Commented=on
  Wheel Omega : Outport
  Requested Motor Torque : Outport  Port=2
  Constrained Motor Torque : Outport  Port=3
  wires:
  Bus Creator/1 -> Wheel Omega/1
  TIRE FORCES (W FRAME)/1 -> Bus Selector/1
  Bus Selector/1 -> [FX_W_FL]  "<FX_W FL>"
  Bus Selector/2 -> [FX_W_FR]  "<FX_W FR>"
  Bus Selector/3 -> [FX_W_RL]  "<FX_W RL>"
  Bus Selector/4 -> [FX_W_RR]  "<FX_W RR>"
  Torque FL/1 -> Switch4/3, Switch4/2
  Bus Creator1/1 -> Requested Motor Torque/1
  ROLLING RESISTANCE (W FRAME)/1 -> Bus Selector1/1
  Bus Selector1/1 -> [F_ROLL_W_FL]  "<F_Roll_FL>"
  Bus Selector1/2 -> [F_ROLL_W_FR]  "<F_Roll_FR>"
  Bus Selector1/3 -> [F_ROLL_W_RL]  "<F_Roll_RL>"
  Bus Selector1/4 -> [F_ROLL_W_RR]  "<F_Roll_RR>"
  Add/1 -> Subsystem4/2(FX Resistance)  "FX Resistance FL"
  Add1/1 -> Subsystem5/2(FX Resistance)  "FX Resistance FR"
  Add2/1 -> Subsystem6/2(FX Resistance)  "FX Resistance RL"
  Add3/1 -> Subsystem7/2(FX Resistance)  "FX Resistance RR"
  Bus Creator2/1 -> Constrained Motor Torque/1
  Data Store Read8/1 -> Switch/2
  Constant4/1 -> Switch/3
  Data Store Read9/1 -> Switch1/2
  Constant5/1 -> Switch1/3
  Data Store Read10/1 -> Switch2/2
  Constant6/1 -> Switch2/3
  Data Store Read11/1 -> Switch3/2
  Constant7/1 -> Switch3/3
  Switch4/1 -> Subsystem4/1(Requested Motor Torque), Bus Creator1/1  "Requested Motor Torque FL"
  Constant8/1 -> Switch4/1
  Constant9/1 -> Switch5/1
  Torque FR/1 -> Switch5/2, Switch5/3
  Switch5/1 -> Subsystem5/1(Requested Motor Torque), Bus Creator1/2  "Requested Motor Torque FR"
  Constant10/1 -> Switch6/1
  Torque RL/1 -> Switch6/2, Switch6/3
  Switch6/1 -> Subsystem6/1(Requested Motor Torque), Bus Creator1/3  "Requested Motor Torque RL"
  Constant11/1 -> Switch7/1
  Torque RR/1 -> Switch7/3, Switch7/2
  Switch7/1 -> Subsystem7/1(Requested Motor Torque), Bus Creator1/4  "Requested Motor Torque RR"
  Bus Selector/5 -> [FY_W_FL]  "<FY_W FL>"
  Bus Selector/6 -> [FY_W_FR]  "<FY_W FR>"
  Bus Selector/7 -> [FY_W_RL]  "<FY_W RL>"
  Bus Selector/8 -> [FY_W_RR]  "<FY_W RR>"
  [FX_W_FL] -> Add/1, Subsystem/1(FX)
  [FX_W_FR] -> Add1/1, Subsystem1/1(FX)
  [FX_W_RL] -> Add2/1, Subsystem2/1(FX)
  [FX_W_RR] -> Add3/1, Subsystem3/1(FX)
  Alpha/1 -> Bus Selector2/1
  Delta_Left/1 -> Abs/1
  Abs/1 -> Sin/1, Cos/1
  Delta_Right/1 -> Abs1/1
  Abs1/1 -> Sin1/1, Cos1/1
  Cos/1 -> [cosDeltaL]
  Cos1/1 -> [cosDeltaR]
  Abs2/1 -> Cos2/1
  Bus Selector2/1 -> Abs6/1, Abs2/1  "<Alpha_RL>"
  Cos2/1 -> [sinAlphaRL]
  Abs3/1 -> Cos3/1
  Bus Selector2/2 -> Abs7/1, Abs3/1  "<Alpha_RR>"
  Cos3/1 -> [sinAlphaRR]
  Subsystem/1(F NET) -> Product/1
  Subsystem1/1(F NET) -> Product1/1
  Subsystem2/1(F NET) -> Product2/1
  Subsystem3/1(F NET) -> Product3/1
  Cos5/1 -> [sinAlphaFR]
  Bus Selector2/4 -> Abs9/1, Abs5/1  "<Alpha_FR>"
  Abs5/1 -> Cos5/1
  Cos4/1 -> [sinAlphaFL]
  Bus Selector2/3 -> Abs8/1, Abs4/1  "<Alpha_FL>"
  Abs4/1 -> Cos4/1
  [FY_W_FL] -> Subsystem/2(FY)
  Sin/1 -> [sinDeltaL]
  Sin1/1 -> [sinDeltaR]
  [FY_W_FR] -> Subsystem1/2(FY)
  [FY_W_RL] -> Subsystem2/2(FY)
  [FY_W_RR] -> Subsystem3/2(FY)
  Cos7/1 -> [cosAlphaRR]
  Abs7/1 -> Cos7/1
  Cos6/1 -> [cosAlphaRL]
  Abs6/1 -> Cos6/1
  [cosAlphaRL] -> Product2/2
  [cosAlphaRR] -> Product3/2
  Product/1 -> Switch/1
  Product1/1 -> Switch1/1
  Product2/1 -> Switch2/1
  Product3/1 -> Switch3/1
  Abs8/1 -> Cos8/1
  Cos8/1 -> [cosAlphaFL]
  Abs9/1 -> Cos9/1
  Cos9/1 -> [cosAlphaFR]
  [cosDeltaL] -> Product/2
  [cosDeltaR] -> Product1/2
  [F_ROLL_W_FL] -> Add/2
  [F_ROLL_W_FR] -> Add1/2
  [F_ROLL_W_RR] -> Add3/2
  [F_ROLL_W_RL] -> Add2/2
  Longitudinal Corner Vel (W Frame)/1 -> Bus Selector3/1
  Bus Selector3/1 -> [Long_Corner_Vel_FL]  "<Longitudinal_Corner_Vel_W FL>"
  Bus Selector3/2 -> [Long_Corner_Vel_FR]  "<Longitudinal_Corner_Vel_W FR>"
  Bus Selector3/3 -> [Long_Corner_Vel_RL]  "<Longitudinal_Corner_Vel_W RL>"
  Bus Selector3/4 -> [Long_Corner_Vel_RR]  "<Longtidutinal_Corner_Vel_W RR>"
  [Long_Corner_Vel_FL] -> Subsystem4/3(Long Corner Vel)
  Subsystem4/2(Constrained Motor Torque) -> Bus Creator2/1  "Constrained Motor Torque FL"
  Subsystem4/1(Wheel Omega) -> Memory/1  "Wheel Omega FL"
  [Long_Corner_Vel_FR] -> Subsystem5/3(Long Corner Vel)
  [Long_Corner_Vel_RL] -> Subsystem6/3(Long Corner Vel)
  [Long_Corner_Vel_RR] -> Subsystem7/3(Long Corner Vel)
  Subsystem5/1(Wheel Omega) -> Memory1/1  "Wheel Omega FR"
  Subsystem6/1(Wheel Omega) -> Memory2/1  "Wheel Omega RL"
  Subsystem7/1(Wheel Omega) -> Memory3/1  "Wheel Omega RR"
  Subsystem5/2(Constrained Motor Torque) -> Bus Creator2/2  "Constrained Motor Torque FR"
  Subsystem6/2(Constrained Motor Torque) -> Bus Creator2/3  "Constrained Motor Torque RL"
  Subsystem7/2(Constrained Motor Torque) -> Bus Creator2/4  "Constrained Motor Torque RR"
  Memory/1 -> Bus Creator/1  "Wheel Omega FL"
  Memory1/1 -> Bus Creator/2  "Wheel Omega FR"
  Memory2/1 -> Bus Creator/3  "Wheel Omega RL"
  Memory3/1 -> Bus Creator/4  "Wheel Omega RR"

== system FullCarLateral/Constant Input PID/Subsystem3 ==
  Vx_B [m/s] : Inport
  Delta [rad] : Inport  Port=2
  Yaw Rate [Rad/s] : Inport  Port=3
  Abs : Abs  SaturateOnIntegerOverflow=off
  Constant : Constant  Value=wb
  Divide : Product  Inputs=**/
  Subtract : Sum  Inputs=+-
  Tan : Trigonometry  Operator=tan
  Yaw Error [rad/s] : Outport
  wires:
  Tan/1 -> Divide/2
  Delta [rad]/1 -> Tan/1
  Constant/1 -> Divide/3
  Subtract/1 -> Yaw Error [rad/s]/1  "Yaw Error [rad/s]"
  Yaw Rate [Rad/s]/1 -> Subtract/2
  Divide/1 -> Subtract/1  "Desired Yaw Rate [rad/s]"
  Abs/1 -> Divide/1
  Vx_B [m/s]/1 -> Abs/1

== system FullCarLateral/Data Input PID/Subsystem3 ==
  Vx_B [m/s] : Inport
  Delta [rad] : Inport  Port=2
  Yaw Rate [Rad/s] : Inport  Port=3
  Abs : Abs  SaturateOnIntegerOverflow=off
  Constant : Constant  Value=wb
  Divide : Product  Inputs=**/
  Subtract : Sum  Inputs=+-
  Tan : Trigonometry  Operator=tan
  Yaw Error [rad/s] : Outport
  wires:
  Vx_B [m/s]/1 -> Abs/1
  Abs/1 -> Divide/1
  Divide/1 -> Subtract/1  "Desired Yaw Rate [rad/s]"
  Yaw Rate [Rad/s]/1 -> Subtract/2
  Subtract/1 -> Yaw Error [rad/s]/1  "Yaw Error [rad/s]"
  Constant/1 -> Divide/3
  Delta [rad]/1 -> Tan/1
  Tan/1 -> Divide/2

== system FullCarLateral/Stop Simulation Based on Distance/If Action Subsystem ==
  In1 : Inport
  Action Port : ActionPort  ActionPortLabel=if(u1 >= u2)
  Out1 : Outport
  wires:
  In1/1 -> Out1/1

== system FullCarLateral/Stop Simulation Based on Distance/If Action Subsystem1 ==
  In1 : Inport
  Action Port : ActionPort  ActionPortLabel=else
  Out1 : Outport
  wires:
  In1/1 -> Out1/1

== system FullCarLateral/Car/Longitudinal Slip/Longitudinal Slip Calc FL ==
  Wheel Omega : Inport
  Requested Motor Torque FL : Inport  Port=2
  Corner Speed : Inport  Port=3
  Accel. Calc : Subsystem  TreatAsAtomicUnit=on
  Brake Calc : Subsystem  TreatAsAtomicUnit=on
  Constant : Constant  Commented=on  Value=R_wheel
  Constant1 : Constant  Value=0
  Constant2 : Constant  Value=R_wheel
  If : If  Commented=on  ElseIfExpressions=u1 < 0
  If Action Subsystem : Subsystem  TreatAsAtomicUnit=on
  If1 : If  IfExpression=u1 >= 0  ElseIfExpressions=u1 < 0
  If2 : If  ElseIfExpressions=u1 < 0
  Merge : Merge  Inputs=3
  Product : Product  Commented=on
  Product1 : Product
  Scope : Scope
  Subtract : Sum  Commented=on  Inputs=+-
  Subtract1 : Sum  Inputs=+-
  SL FL : Outport
  wires:
  Wheel Omega/1 -> Product1/1, Brake Calc/1(Wheel Omega), Accel. Calc/2(Wheel Omega1)
  Accel. Calc/1(SL) -> Merge/1
  Corner Speed/1 -> Subtract1/2, Accel. Calc/1(Corner Speed), Brake Calc/2(Corner Speed)
  Brake Calc/1(SL) -> Merge/2
  Merge/1 -> SL FL/1  "SL"
  Constant/1 -> Product/2
  Subtract/1 -> If/1
  Product/1 -> Subtract/1
  Requested Motor Torque FL/1 -> If1/1
  Constant2/1 -> Product1/2
  Product1/1 -> Subtract1/1, Scope/1
  Subtract1/1 -> If2/1
  If2/1 -> Accel. Calc/Action
  If2/2 -> Brake Calc/Action
  If2/3 -> If Action Subsystem/Action
  Constant1/1 -> If Action Subsystem/1(in)
  If Action Subsystem/1(Out1) -> Merge/3

== system FullCarLateral/Car/Longitudinal Slip/Longitudinal Slip Calc FL1 ==
  Wheel Omega : Inport
  Requested Motor Torque FL : Inport  Port=2
  Corner Speed : Inport  Port=3
  Accel. Calc : Subsystem  TreatAsAtomicUnit=on
  Brake Calc : Subsystem  TreatAsAtomicUnit=on
  Constant : Constant  Commented=on  Value=R_wheel
  Constant1 : Constant  Value=0
  Constant2 : Constant  Value=R_wheel
  If : If  Commented=on  ElseIfExpressions=u1 < 0
  If Action Subsystem : Subsystem  TreatAsAtomicUnit=on
  If1 : If  IfExpression=u1 >= 0  ElseIfExpressions=u1 < 0
  If2 : If  ElseIfExpressions=u1 < 0
  Merge : Merge  Inputs=3
  Product : Product  Commented=on
  Product1 : Product
  Scope : Scope
  Subtract : Sum  Commented=on  Inputs=+-
  Subtract1 : Sum  Inputs=+-
  SL FL : Outport
  wires:
  If Action Subsystem/1(Out1) -> Merge/3
  Constant1/1 -> If Action Subsystem/1(Corner Speed)
  If2/3 -> If Action Subsystem/Action
  If2/2 -> Brake Calc/Action
  If2/1 -> Accel. Calc/Action
  Subtract1/1 -> If2/1
  Product1/1 -> Scope/1, Subtract1/1
  Constant2/1 -> Product1/2
  Requested Motor Torque FL/1 -> If1/1
  Product/1 -> Subtract/1
  Subtract/1 -> If/1
  Constant/1 -> Product/2
  Merge/1 -> SL FL/1  "SL"
  Brake Calc/1(SL) -> Merge/2
  Corner Speed/1 -> Brake Calc/2(Corner Speed), Accel. Calc/1(Corner Speed), Subtract1/2
  Accel. Calc/1(SL) -> Merge/1
  Wheel Omega/1 -> Accel. Calc/2(Wheel Omega1), Brake Calc/1(Wheel Omega), Product1/1

== system FullCarLateral/Car/Longitudinal Slip/Longitudinal Slip Calc FL2 ==
  Wheel Omega : Inport
  Requested Motor Torque FL : Inport  Port=2
  Corner Speed : Inport  Port=3
  Accel. Calc : Subsystem  TreatAsAtomicUnit=on
  Brake Calc : Subsystem  TreatAsAtomicUnit=on
  Constant : Constant  Commented=on  Value=R_wheel
  Constant1 : Constant  Value=0
  Constant2 : Constant  Value=R_wheel
  If : If  Commented=on  ElseIfExpressions=u1 < 0
  If Action Subsystem : Subsystem  TreatAsAtomicUnit=on
  If1 : If  IfExpression=u1 >= 0  ElseIfExpressions=u1 < 0
  If2 : If  ElseIfExpressions=u1 < 0
  Merge : Merge  Inputs=3
  Product : Product  Commented=on
  Product1 : Product
  Scope : Scope
  Subtract : Sum  Commented=on  Inputs=+-
  Subtract1 : Sum  Inputs=+-
  SL FL : Outport
  wires:
  Wheel Omega/1 -> Product1/1, Brake Calc/1(Wheel Omega), Accel. Calc/2(Wheel Omega1)
  Accel. Calc/1(SL) -> Merge/1
  Corner Speed/1 -> Subtract1/2, Accel. Calc/1(Corner Speed), Brake Calc/2(Corner Speed)
  Brake Calc/1(SL) -> Merge/2
  Merge/1 -> SL FL/1  "SL"
  Constant/1 -> Product/2
  Subtract/1 -> If/1
  Product/1 -> Subtract/1
  Requested Motor Torque FL/1 -> If1/1
  Constant2/1 -> Product1/2
  Product1/1 -> Subtract1/1, Scope/1
  Subtract1/1 -> If2/1
  If2/1 -> Accel. Calc/Action
  If2/2 -> Brake Calc/Action
  If2/3 -> If Action Subsystem/Action
  Constant1/1 -> If Action Subsystem/1(Corner Speed)
  If Action Subsystem/1(Out1) -> Merge/3

== system FullCarLateral/Car/Longitudinal Slip/Longitudinal Slip Calc FL3 ==
  Wheel Omega : Inport
  Requested Motor Torque FL : Inport  Port=2
  Corner Speed : Inport  Port=3
  Accel. Calc : Subsystem  TreatAsAtomicUnit=on
  Brake Calc : Subsystem  TreatAsAtomicUnit=on
  Constant : Constant  Commented=on  Value=R_wheel
  Constant1 : Constant  Value=0
  Constant2 : Constant  Value=R_wheel
  If : If  Commented=on  ElseIfExpressions=u1 < 0
  If Action Subsystem : Subsystem  TreatAsAtomicUnit=on
  If1 : If  IfExpression=u1 >= 0  ElseIfExpressions=u1 < 0
  If2 : If  ElseIfExpressions=u1 < 0
  Merge : Merge  Inputs=3
  Product : Product  Commented=on
  Product1 : Product
  Scope : Scope
  Subtract : Sum  Commented=on  Inputs=+-
  Subtract1 : Sum  Inputs=+-
  SL FL : Outport
  wires:
  If Action Subsystem/1(Out1) -> Merge/3
  Constant1/1 -> If Action Subsystem/1(Corner Speed)
  If2/3 -> If Action Subsystem/Action
  If2/2 -> Brake Calc/Action
  If2/1 -> Accel. Calc/Action
  Subtract1/1 -> If2/1
  Product1/1 -> Scope/1, Subtract1/1
  Constant2/1 -> Product1/2
  Requested Motor Torque FL/1 -> If1/1
  Product/1 -> Subtract/1
  Subtract/1 -> If/1
  Constant/1 -> Product/2
  Merge/1 -> SL FL/1  "SL"
  Brake Calc/1(SL) -> Merge/2
  Corner Speed/1 -> Brake Calc/2(Corner Speed), Accel. Calc/1(Corner Speed), Subtract1/2
  Accel. Calc/1(SL) -> Merge/1
  Wheel Omega/1 -> Accel. Calc/2(Wheel Omega1), Brake Calc/1(Wheel Omega), Product1/1

== system FullCarLateral/Car/Steering Kinematics/Ackerman Calculation ==
  Delta Avg : Inport
  Action Port : ActionPort  ActionPortLabel=if(u1 ~= 0)
  Add : Sum
  Atan : Trigonometry  Operator=atan
  Atan1 : Trigonometry  Operator=atan
  Constant : Constant  Value=wb
  Constant1 : Constant  Value=trackWidth
  Degrees to Radians : simulink_extras/Transformations/Degrees to Radians
  Divide : Product  Inputs=*/
  Divide1 : Product  Inputs=*/
  Fcn : Fcn  Expr=1/u
  Multiply : Gain  Gain=0.5
  Product : Product
  Subtract : Sum  Inputs=+-
  Tan : Trigonometry  Operator=tan
  Delta Left : Outport
  Delta Right : Outport  Port=2
  wires:
  Delta Avg/1 -> Degrees to Radians/1
  Fcn/1 -> Product/2  "cot(u)"
  Tan/1 -> Fcn/1
  Constant/1 -> Divide1/1, Product/1, Divide/1
  Constant1/1 -> Multiply/1
  Degrees to Radians/1 -> Tan/1
  Divide/1 -> Atan/1
  Atan1/1 -> Delta Right/1
  Divide1/1 -> Atan1/1
  Add/1 -> Divide1/2
  Product/1 -> Add/1, Subtract/1
  Atan/1 -> Delta Left/1
  Subtract/1 -> Divide/2
  Multiply/1 -> Add/2, Subtract/2

== system FullCarLateral/Car/Tire Model Pacejka 5.2/FY DIRECTIONAL CONSTRAIN FL ==
  FY : Inport
  SA : Inport  Port=2
  Constant : Constant  Value=0
  If : If  IfExpression=u1 < 0  ElseIfExpressions=u1 > 0
  If Action Subsystem : Subsystem  TreatAsAtomicUnit=on
  Merge : Merge  Inputs=3
  NEGATIVE FY : Subsystem  TreatAsAtomicUnit=on
  POSITIVE FY : Subsystem  TreatAsAtomicUnit=on
  FY DIR CONSTRAINED : Outport
  wires:
  FY/1 -> NEGATIVE FY/1(In1), POSITIVE FY/1(In1)
  POSITIVE FY/1(Out1) -> Merge/2
  If/1 -> POSITIVE FY/Action  "NEGATIVE SA"
  NEGATIVE FY/1(Out1) -> Merge/1
  SA/1 -> If/1
  Merge/1 -> FY DIR CONSTRAINED/1
  If/2 -> NEGATIVE FY/Action  "POSITIVE SA"
  If/3 -> If Action Subsystem/Action
  Constant/1 -> If Action Subsystem/1(In1)
  If Action Subsystem/1(Out1) -> Merge/3

== system FullCarLateral/Car/Tire Model Pacejka 5.2/FY DIRECTIONAL CONSTRAIN FR ==
  FY : Inport
  SA : Inport  Port=2
  Constant : Constant  Value=0
  If : If  IfExpression=u1 < 0  ElseIfExpressions=u1 > 0
  If Action Subsystem : Subsystem  TreatAsAtomicUnit=on
  Merge : Merge  Inputs=3
  NEGATIVE FY : Subsystem  TreatAsAtomicUnit=on
  POSITIVE FY : Subsystem  TreatAsAtomicUnit=on
  FY DIR CONSTRAINED : Outport
  wires:
  If Action Subsystem/1(Out1) -> Merge/3
  Constant/1 -> If Action Subsystem/1(In1)
  If/3 -> If Action Subsystem/Action
  If/2 -> NEGATIVE FY/Action  "POSITIVE SA"
  Merge/1 -> FY DIR CONSTRAINED/1
  SA/1 -> If/1
  NEGATIVE FY/1(Out1) -> Merge/1
  If/1 -> POSITIVE FY/Action  "NEGATIVE SA"
  POSITIVE FY/1(Out1) -> Merge/2
  FY/1 -> POSITIVE FY/1(In1), NEGATIVE FY/1(In1)

== system FullCarLateral/Car/Tire Model Pacejka 5.2/FY DIRECTIONAL CONSTRAIN RL ==
  FY : Inport
  SA : Inport  Port=2
  SA FL : Inport  Port=3
  Abs : Abs  SaturateOnIntegerOverflow=off
  Constant : Constant  Value=0
  Constant1 : Constant  Value=0
  If : If  IfExpression=u1 < 0  ElseIfExpressions=u1 > 0
  If Action Subsystem : Subsystem  TreatAsAtomicUnit=on
  Merge : Merge  Inputs=3
  NEGATIVE FY : Subsystem  TreatAsAtomicUnit=on
  POSITIVE FY : Subsystem  TreatAsAtomicUnit=on
  Switch : Switch  Criteria=u2 > Threshold  Threshold=0.25  SaturateOnIntegerOverflow=off  InputSameDT=off
  FY DIR CONSTRAINED : Outport
  wires:
  FY/1 -> NEGATIVE FY/1(In1), POSITIVE FY/1(In1)
  POSITIVE FY/1(Out1) -> Merge/2
  If/1 -> POSITIVE FY/Action  "NEGATIVE SA"
  NEGATIVE FY/1(Out1) -> Merge/1
  SA/1 -> If/1
  If/2 -> NEGATIVE FY/Action  "POSITIVE SA"
  If/3 -> If Action Subsystem/Action
  Constant/1 -> If Action Subsystem/1(In1)
  If Action Subsystem/1(Out1) -> Merge/3
  Constant1/1 -> Switch/3
  SA FL/1 -> Abs/1
  Abs/1 -> Switch/2
  Merge/1 -> FY DIR CONSTRAINED/1

== system FullCarLateral/Car/Tire Model Pacejka 5.2/FY DIRECTIONAL CONSTRAIN RR ==
  FY : Inport
  SA : Inport  Port=2
  SA FR : Inport  Port=3
  Abs : Abs  SaturateOnIntegerOverflow=off
  Constant : Constant  Value=0
  Constant1 : Constant  Value=0
  If : If  IfExpression=u1 < 0  ElseIfExpressions=u1 > 0
  If Action Subsystem : Subsystem  TreatAsAtomicUnit=on
  Merge : Merge  Inputs=3
  NEGATIVE FY : Subsystem  TreatAsAtomicUnit=on
  POSITIVE FY : Subsystem  TreatAsAtomicUnit=on
  Switch : Switch  Criteria=u2 > Threshold  Threshold=0.25  SaturateOnIntegerOverflow=off  InputSameDT=off
  FY DIR CONSTRAINED : Outport
  wires:
  If Action Subsystem/1(Out1) -> Merge/3
  Constant/1 -> If Action Subsystem/1(In1)
  If/3 -> If Action Subsystem/Action
  If/2 -> NEGATIVE FY/Action  "POSITIVE SA"
  SA/1 -> If/1
  NEGATIVE FY/1(Out1) -> Merge/1
  If/1 -> POSITIVE FY/Action  "NEGATIVE SA"
  POSITIVE FY/1(Out1) -> Merge/2
  FY/1 -> POSITIVE FY/1(In1), NEGATIVE FY/1(In1)
  Constant1/1 -> Switch/3
  SA FR/1 -> Abs/1
  Abs/1 -> Switch/2
  Merge/1 -> FY DIR CONSTRAINED/1

== system FullCarLateral/Car/Tire Model Pacejka 5.2/Subsystem ==
  FX : Inport
  If : If  IfExpression=u1 >= 0
  If Action Subsystem : Subsystem  TreatAsAtomicUnit=on
  If Action Subsystem1 : Subsystem  TreatAsAtomicUnit=on
  Merge : Merge
  FX_W FL : Outport
  wires:
  If/1 -> If Action Subsystem/Action
  FX/1 -> If/1, If Action Subsystem1/1(FX), If Action Subsystem/1(FX)
  Merge/1 -> FX_W FL/1  "FX_W FL"
  If/2 -> If Action Subsystem1/Action
  If Action Subsystem/1(Out1) -> Merge/1
  If Action Subsystem1/1(Out1) -> Merge/2
